simulink library "blocklib"  (R2019b)
settings: Solver=VariableStepAuto  StartTime=0.0  StopTime=10.0  RelTol=1e-3
undefined symbols (not defined in the file or in its folder): magnitude
libraries: $bdroot x11
settings Model: Creator=Imanol  LastModifiedBy=imanol
settings SFSimCC: CustomCodeUndefinedFunction=UseInterfaceOnly

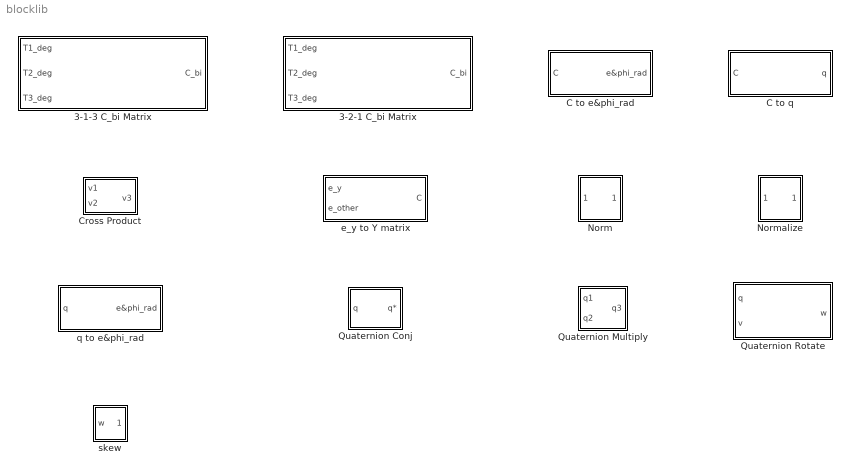
== system blocklib ==
  3-1-3 C_bi Matrix : Subsystem  Tag=|
      | text(.05,.5,'{\itEquation:}  \Sigma \alpha^2 + 
      | \beta^2 \rightarrow \infty, \Pi, \phi_3 = {\bfcool}', 
      | 'hor','left','texmode','on')
      mask Display: text(.5,.5,'R_z^T(\theta_3)\cdot R_x^T(\theta_2)\cdot R_z^T(\theta_1)', 'hor','center','texmode','on')
  3-2-1 C_bi Matrix : Subsystem  Tag=|
      | text(.05,.5,'{\itEquation:}  \Sigma \alpha^2 + 
      | \beta^2 \rightarrow \infty, \Pi, \phi_3 = {\bfcool}', 
      | 'hor','left','texmode','on')
      mask Display: text(.5,.5,'R_x^T(\theta_3)\cdot R_y^T(\theta_2)\cdot R_z^T(\theta_1)', 'hor','center','texmode','on')
  C to e&phi_rad : Subsystem
      mask Display: text(.5,.5,'C\rightarrow [{\bf e}; phi_{rad}]', 'hor','center','texmode','on')
  C to q : Subsystem
      mask Display: text(.5,.5,'C\rightarrow [{\bf q}; q_4]', 'hor','center','texmode','on')
  Cross Product : Subsystem
      mask Display: text(.5,.5,'{\bf v_1} \times {\bf v_2}', 'hor','center','texmode','on')
  Norm : Subsystem
      mask Display: text(.5,.5,'|{\bf u}|', 'hor','center','texmode','on')
  Normalize : Subsystem
      mask Display: text(.5,.5,'{\bf u}/|{\bf u}|', 'hor','center','texmode','on')
  Quaternion Conj : Subsystem
      mask Display: text(.5,.5,'Conj(q)', 'hor','center','texmode','on')
  Quaternion Multiply : Subsystem
      mask Display: text(.5,.5,'q_1\times q_2', 'hor','center','texmode','on')
  Quaternion Rotate : Subsystem
      mask Display: text(.5,.5,'q \times [{\bf v}; 0] \times q^*', 'hor','center','texmode','on')
  e_y to Y matrix : Subsystem
      mask Display: text(.5,.5,'[0;1;0]=C\cdot{\bf e_y}','hor','center', 'texmode','on')
  q to e&phi_rad : Subsystem
      mask Display: text(.5,.5,'q\rightarrow [{\bf e}; phi_{rad}]', 'hor','center','texmode','on')
  skew : Subsystem
      mask Display: text(.5,.5,'w^x', 'hor','center','texmode','on')

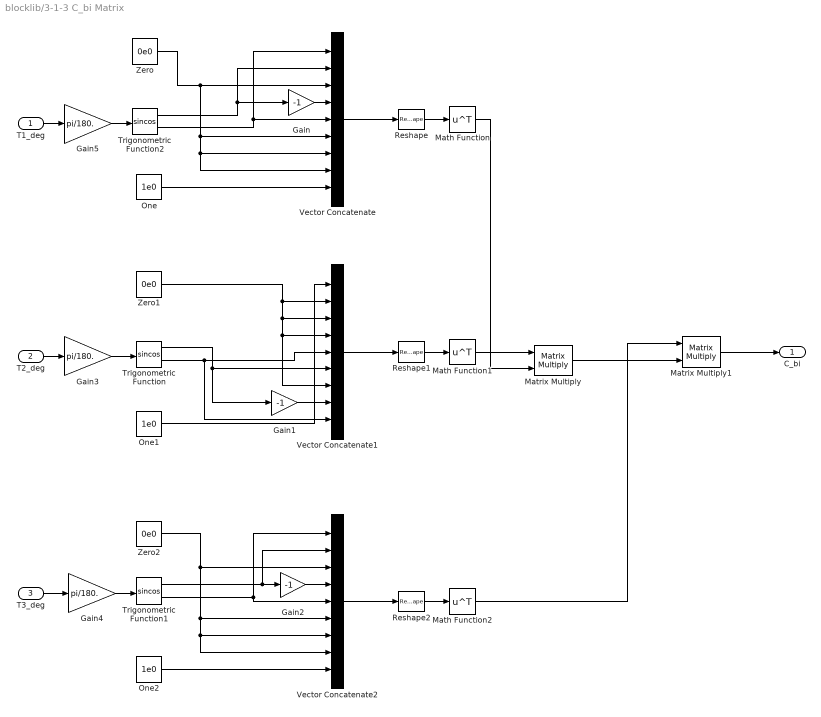
== system blocklib/3-1-3 C_bi Matrix ==
  T1_deg : Inport
  T2_deg : Inport  Port=2
  T3_deg : Inport  Port=3
  Gain : Gain  Gain=-1
  Gain1 : Gain  Gain=-1
  Gain2 : Gain  Gain=-1
  Gain3 : Gain  Gain=pi/180.
  Gain4 : Gain  Gain=pi/180.
  Gain5 : Gain  Gain=pi/180.
  Math Function : Math  Operator=transpose  SignedPower=off  SaturateOnIntegerOverflow=on
  Math Function1 : Math  Operator=transpose  SignedPower=off  SaturateOnIntegerOverflow=on
  Math Function2 : Math  Operator=transpose  SignedPower=off  SaturateOnIntegerOverflow=on
  Matrix Multiply : Product  Multiplication=Matrix(*)
  Matrix Multiply1 : Product  Multiplication=Matrix(*)
  One : Constant  Value=1e0
  One1 : Constant  Value=1e0
  One2 : Constant  Value=1e0
  Reshape : Reshape  OutputDimensionality=Customize  OutputDimensions=[3,3]
  Reshape1 : Reshape  OutputDimensionality=Customize  OutputDimensions=[3,3]
  Reshape2 : Reshape  OutputDimensionality=Customize  OutputDimensions=[3,3]
  Trigonometric Function : Trigonometry  Operator=sincos
  Trigonometric Function1 : Trigonometry  Operator=sincos
  Trigonometric Function2 : Trigonometry  Operator=sincos
  Vector Concatenate : Concatenate  NumInputs=9
  Vector Concatenate1 : Concatenate  NumInputs=9
  Vector Concatenate2 : Concatenate  NumInputs=9
  Zero : Constant  Value=0e0
  Zero1 : Constant  Value=0e0
  Zero2 : Constant  Value=0e0
  C_bi : Outport
  wires:
  T3_deg/1 -> Gain4/1
  T2_deg/1 -> Gain3/1
  Trigonometric Function2/2 -> Vector Concatenate/5, Vector Concatenate/1
  Trigonometric Function2/1 -> Gain/1, Vector Concatenate/2
  Zero/1 -> Vector Concatenate/7, Vector Concatenate/8, Vector Concatenate/6, Vector Concatenate/3
  Gain/1 -> Vector Concatenate/4
  One/1 -> Vector Concatenate/9
  Vector Concatenate/1 -> Reshape/1
  Vector Concatenate1/1 -> Reshape1/1
  One1/1 -> Vector Concatenate1/1
  Zero1/1 -> Vector Concatenate1/7, Vector Concatenate1/4, Vector Concatenate1/3, Vector Concatenate1/2
  Trigonometric Function/2 -> Vector Concatenate1/9, Vector Concatenate1/5
  Trigonometric Function/1 -> Gain1/1, Vector Concatenate1/6
  Gain1/1 -> Vector Concatenate1/8
  Trigonometric Function1/1 -> Vector Concatenate2/2, Gain2/1
  One2/1 -> Vector Concatenate2/9
  Gain2/1 -> Vector Concatenate2/4
  Trigonometric Function1/2 -> Vector Concatenate2/5, Vector Concatenate2/1
  Zero2/1 -> Vector Concatenate2/7, Vector Concatenate2/8, Vector Concatenate2/6, Vector Concatenate2/3
  Reshape1/1 -> Math Function1/1
  Reshape/1 -> Math Function/1
  Matrix Multiply/1 -> Matrix Multiply1/2
  Reshape2/1 -> Math Function2/1
  Matrix Multiply1/1 -> C_bi/1
  Vector Concatenate2/1 -> Reshape2/1
  Gain4/1 -> Trigonometric Function1/1
  Gain3/1 -> Trigonometric Function/1
  T1_deg/1 -> Gain5/1
  Gain5/1 -> Trigonometric Function2/1
  Math Function/1 -> Matrix Multiply/2
  Math Function1/1 -> Matrix Multiply/1
  Math Function2/1 -> Matrix Multiply1/1

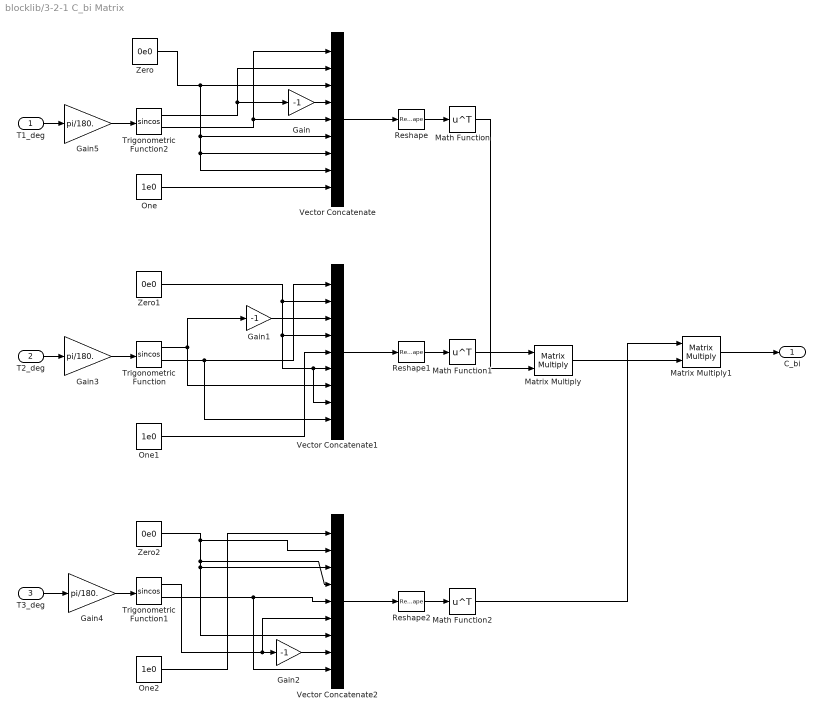
== system blocklib/3-2-1 C_bi Matrix ==
  T1_deg : Inport
  T2_deg : Inport  Port=2
  T3_deg : Inport  Port=3
  Gain : Gain  Gain=-1
  Gain1 : Gain  Gain=-1
  Gain2 : Gain  Gain=-1
  Gain3 : Gain  Gain=pi/180.
  Gain4 : Gain  Gain=pi/180.
  Gain5 : Gain  Gain=pi/180.
  Math Function : Math  Operator=transpose  SignedPower=off  SaturateOnIntegerOverflow=on
  Math Function1 : Math  Operator=transpose  SignedPower=off  SaturateOnIntegerOverflow=on
  Math Function2 : Math  Operator=transpose  SignedPower=off  SaturateOnIntegerOverflow=on
  Matrix Multiply : Product  Multiplication=Matrix(*)
  Matrix Multiply1 : Product  Multiplication=Matrix(*)
  One : Constant  Value=1e0
  One1 : Constant  Value=1e0
  One2 : Constant  Value=1e0
  Reshape : Reshape  OutputDimensionality=Customize  OutputDimensions=[3,3]
  Reshape1 : Reshape  OutputDimensionality=Customize  OutputDimensions=[3,3]
  Reshape2 : Reshape  OutputDimensionality=Customize  OutputDimensions=[3,3]
  Trigonometric Function : Trigonometry  Operator=sincos
  Trigonometric Function1 : Trigonometry  Operator=sincos
  Trigonometric Function2 : Trigonometry  Operator=sincos
  Vector Concatenate : Concatenate  NumInputs=9
  Vector Concatenate1 : Concatenate  NumInputs=9
  Vector Concatenate2 : Concatenate  NumInputs=9
  Zero : Constant  Value=0e0
  Zero1 : Constant  Value=0e0
  Zero2 : Constant  Value=0e0
  C_bi : Outport
  wires:
  T3_deg/1 -> Gain4/1
  T2_deg/1 -> Gain3/1
  Trigonometric Function2/2 -> Vector Concatenate/5, Vector Concatenate/1
  Trigonometric Function2/1 -> Gain/1, Vector Concatenate/2
  Zero/1 -> Vector Concatenate/7, Vector Concatenate/8, Vector Concatenate/6, Vector Concatenate/3
  Gain/1 -> Vector Concatenate/4
  One/1 -> Vector Concatenate/9
  Vector Concatenate/1 -> Reshape/1
  Vector Concatenate1/1 -> Reshape1/1
  One1/1 -> Vector Concatenate1/5
  Zero1/1 -> Vector Concatenate1/2, Vector Concatenate1/8, Vector Concatenate1/6, Vector Concatenate1/4
  Trigonometric Function/2 -> Vector Concatenate1/1, Vector Concatenate1/9
  Trigonometric Function/1 -> Gain1/1, Vector Concatenate1/7
  Gain1/1 -> Vector Concatenate1/3
  Trigonometric Function1/1 -> Vector Concatenate2/6, Gain2/1
  One2/1 -> Vector Concatenate2/1
  Gain2/1 -> Vector Concatenate2/8
  Trigonometric Function1/2 -> Vector Concatenate2/9, Vector Concatenate2/5
  Zero2/1 -> Vector Concatenate2/2, Vector Concatenate2/7, Vector Concatenate2/3, Vector Concatenate2/4
  Reshape1/1 -> Math Function1/1
  Reshape/1 -> Math Function/1
  Matrix Multiply/1 -> Matrix Multiply1/2
  Reshape2/1 -> Math Function2/1
  Matrix Multiply1/1 -> C_bi/1
  Vector Concatenate2/1 -> Reshape2/1
  Gain4/1 -> Trigonometric Function1/1
  Gain3/1 -> Trigonometric Function/1
  T1_deg/1 -> Gain5/1
  Math Function/1 -> Matrix Multiply/2
  Math Function1/1 -> Matrix Multiply/1
  Math Function2/1 -> Matrix Multiply1/1
  Gain5/1 -> Trigonometric Function2/1

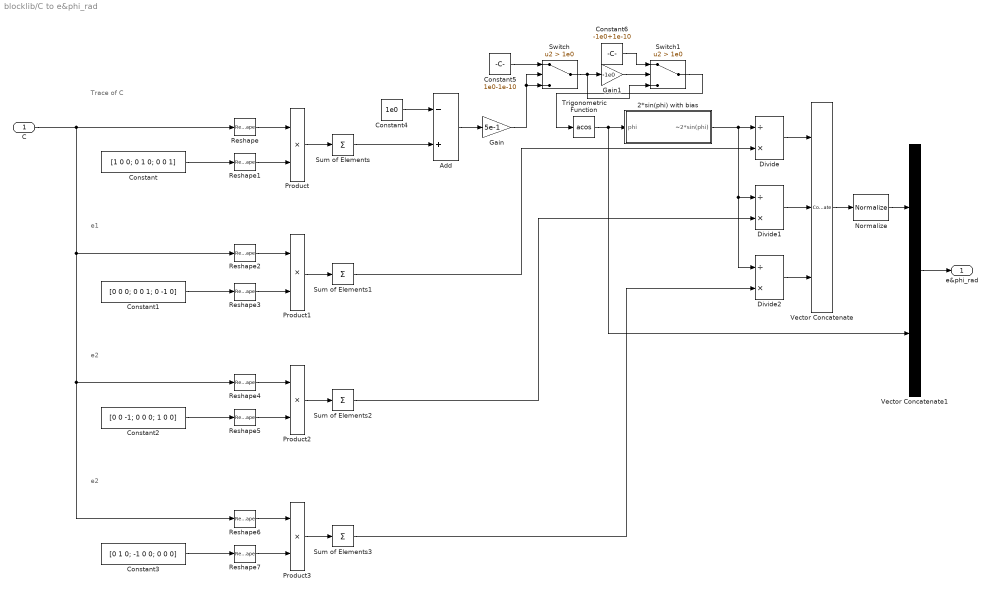
== system blocklib/C to e&phi_rad ==
  note: Trace of C
  note: e1
  note: e2
  note: e2
  C : Inport
  2*sin(phi) with bias : Subsystem
  Add : Sum  Inputs=-+
  Constant : Constant  Value=[1 0 0; 0 1 0; 0 0 1]
  Constant1 : Constant  Value=[0 0 0; 0 0 1; 0 -1 0]
  Constant2 : Constant  Value=[0 0 -1; 0 0 0; 1 0 0]
  Constant3 : Constant  Value=[0 1 0; -1 0 0; 0 0 0]
  Constant4 : Constant  Value=1e0
  Constant5 : Constant  Value=1e0-1e-10
  Constant6 : Constant  Value=-1e0+1e-10
  Divide : Product  Inputs=/*
  Divide1 : Product  Inputs=/*
  Divide2 : Product  Inputs=/*
  Gain : Gain  Gain=5e-1
  Gain1 : Gain  Gain=-1e0
  Normalize : $bdroot/Normalize  SystemSampleTime=-1  Latency=0  AutoFrameSizeCalculation=off
  Product{,1..3} (4 alike) : Product
  Reshape{,1..7} (8 alike) : Reshape  OutputDimensionality=Customize  OutputDimensions=[9,1]
  Sum of Elements{,1..3} (4 alike) : Sum  Inputs=+
  Switch : Switch  Criteria=u2 > Threshold  Threshold=1e0  ZeroCross=off
  Switch1 : Switch  Criteria=u2 > Threshold  Threshold=1e0  ZeroCross=off
  Trigonometric Function : Trigonometry  Operator=acos  OutputSignalType=real
  Vector Concatenate : Concatenate  NumInputs=3
  Vector Concatenate1 : Concatenate
  e&phi_rad : Outport
  wires:
  Switch1/1 -> Trigonometric Function/1
  Constant6/1 -> Switch1/1
  Switch/1 -> Gain1/1, Switch1/3
  Gain1/1 -> Switch1/2
  Constant5/1 -> Switch/1
  Gain/1 -> Switch/2, Switch/3
  Constant/1 -> Reshape1/1
  Reshape1/1 -> Product/2
  Reshape/1 -> Product/1
  Product/1 -> Sum of Elements/1
  Reshape2/1 -> Product1/1
  Product1/1 -> Sum of Elements1/1
  Constant1/1 -> Reshape3/1
  Reshape3/1 -> Product1/2
  Reshape5/1 -> Product2/2
  Constant2/1 -> Reshape5/1
  Product2/1 -> Sum of Elements2/1
  Reshape4/1 -> Product2/1
  Reshape7/1 -> Product3/2
  Reshape6/1 -> Product3/1
  Constant3/1 -> Reshape7/1
  C/1 -> Reshape6/1, Reshape4/1, Reshape2/1, Reshape/1
  Product3/1 -> Sum of Elements3/1
  Sum of Elements/1 -> Add/2
  Constant4/1 -> Add/1
  Add/1 -> Gain/1
  Sum of Elements1/1 -> Divide/2
  Sum of Elements2/1 -> Divide1/2
  Sum of Elements3/1 -> Divide2/2
  Divide/1 -> Vector Concatenate/1
  Divide1/1 -> Vector Concatenate/2
  Divide2/1 -> Vector Concatenate/3
  2*sin(phi) with bias/1(~2*sin(phi)) -> Divide/1, Divide2/1, Divide1/1
  Vector Concatenate1/1 -> e&phi_rad/1
  Vector Concatenate/1 -> Normalize/1
  Trigonometric Function/1 -> Vector Concatenate1/2, 2*sin(phi) with bias/1(phi)
  Normalize/1 -> Vector Concatenate1/1

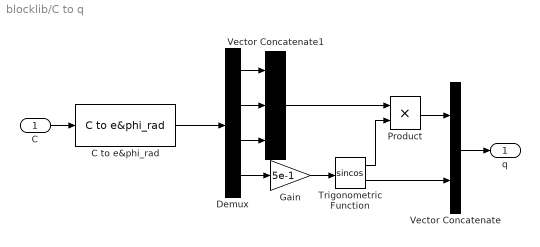
== system blocklib/C to q ==
  C : Inport
  C to e&phi_rad : $bdroot/C to e&phi_rad  SystemSampleTime=-1  Latency=0  AutoFrameSizeCalculation=off
  Demux : Demux
  Gain : Gain  Gain=5e-1
  Product : Product
  Trigonometric Function : Trigonometry  Operator=sincos
  Vector Concatenate : Concatenate
  Vector Concatenate1 : Concatenate  NumInputs=3
  q : Outport
  wires:
  Trigonometric Function/2 -> Vector Concatenate/2
  Demux/3 -> Vector Concatenate1/3
  Demux/4 -> Gain/1
  Demux/2 -> Vector Concatenate1/2
  Vector Concatenate1/1 -> Product/1
  Demux/1 -> Vector Concatenate1/1
  Trigonometric Function/1 -> Product/2
  Product/1 -> Vector Concatenate/1
  Vector Concatenate/1 -> q/1
  Gain/1 -> Trigonometric Function/1
  C/1 -> C to e&phi_rad/1
  C to e&phi_rad/1 -> Demux/1

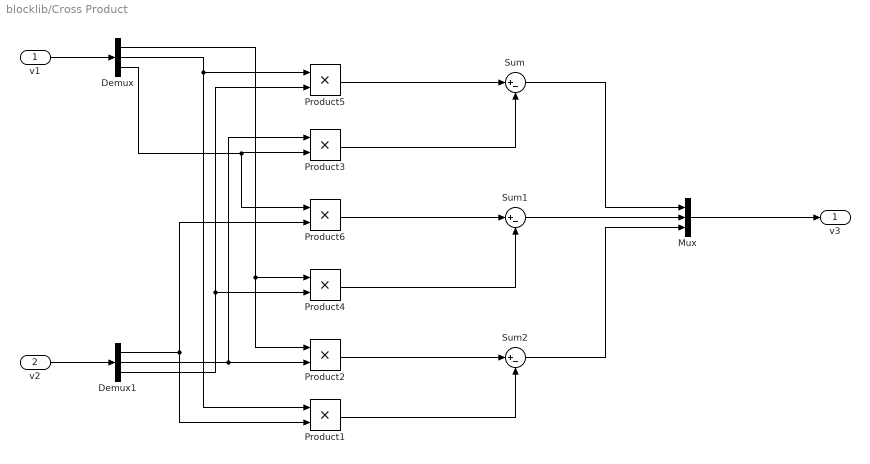
== system blocklib/Cross Product ==
  v1 : Inport
  v2 : Inport  Port=2
  Demux : Demux  Outputs=3
  Demux1 : Demux  Outputs=3
  Mux : Mux  Inputs=3
  Product{1..6} (6 alike) : Product
  Sum : Sum  Inputs=|+-
  Sum1 : Sum  Inputs=|+-
  Sum2 : Sum  Inputs=|+-
  v3 : Outport  VectorParamsAs1DForOutWhenUnconnected=off
  wires:
  Demux/3 -> Product6/1, Product3/2
  Product1/1 -> Sum2/2
  Product2/1 -> Sum2/1
  Product3/1 -> Sum/2
  v2/1 -> Demux1/1
  Demux/2 -> Product1/1, Product5/1
  Demux/1 -> Product2/1, Product4/1
  Product5/1 -> Sum/1
  Demux1/3 -> Product5/2, Product4/2
  Product4/1 -> Sum1/2
  Sum1/1 -> Mux/2
  Sum2/1 -> Mux/3
  v1/1 -> Demux/1
  Demux1/1 -> Product6/2, Product1/2
  Product6/1 -> Sum1/1
  Mux/1 -> v3/1
  Sum/1 -> Mux/1
  Demux1/2 -> Product3/1, Product2/2

== system blocklib/Norm ==
  In1 : Inport
  Math Function : Math  Operator=magnitude^2  SignedPower=off  SaturateOnIntegerOverflow=on
  Sqrt : Sqrt  SaturateOnIntegerOverflow=on
  Sum of Elements : Sum  Inputs=+
  Out1 : Outport
  wires:
  In1/1 -> Math Function/1
  Sum of Elements/1 -> Sqrt/1
  Math Function/1 -> Sum of Elements/1
  Sqrt/1 -> Out1/1

== system blocklib/Normalize ==
  In1 : Inport
  Divide : Product  Inputs=*/
  Math Function : Math  Operator=magnitude^2  SignedPower=off  SaturateOnIntegerOverflow=on
  One : Constant
  Sqrt : Sqrt  SaturateOnIntegerOverflow=on
  Sum of Elements : Sum  Inputs=+
  Switch : Switch  Criteria=u2 > Threshold
  Out1 : Outport
  wires:
  In1/1 -> Divide/1, Math Function/1
  Sqrt/1 -> Switch/1, Switch/2
  Sum of Elements/1 -> Sqrt/1
  Math Function/1 -> Sum of Elements/1
  Divide/1 -> Out1/1
  Switch/1 -> Divide/2
  One/1 -> Switch/3

== system blocklib/Quaternion Conj ==
  q : Inport
  Demux1 : Demux
  Gain : Gain  Gain=-1e0
  Mux1 : Mux  Inputs=3
  Vector Concatenate : Concatenate
  q* : Outport  VectorParamsAs1DForOutWhenUnconnected=off
  wires:
  q/1 -> Demux1/1
  Demux1/1 -> Mux1/1
  Demux1/2 -> Mux1/2
  Demux1/3 -> Mux1/3
  Mux1/1 -> Gain/1
  Gain/1 -> Vector Concatenate/1
  Vector Concatenate/1 -> q*/1
  Demux1/4 -> Vector Concatenate/2

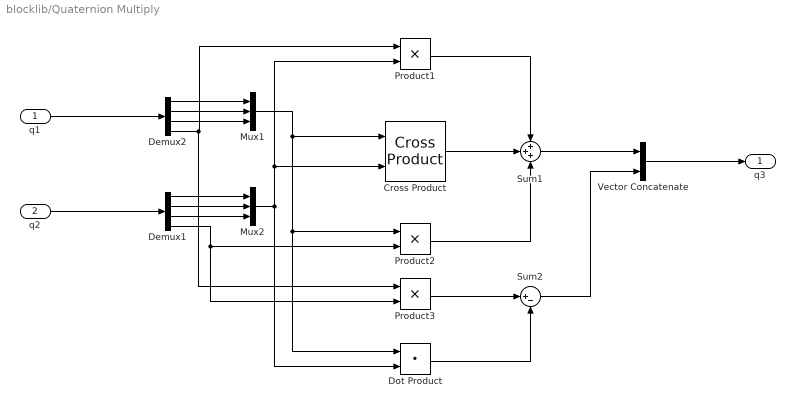
== system blocklib/Quaternion Multiply ==
  q1 : Inport
  q2 : Inport  Port=2
  Cross Product : $bdroot/Cross Product  SystemSampleTime=-1  Latency=0  AutoFrameSizeCalculation=off
  Demux1 : Demux
  Demux2 : Demux
  Dot Product : DotProduct  InputSameDT=on  OutDataTypeStr=Inherit: Inherit via internal rule
  Mux1 : Mux  Inputs=3
  Mux2 : Mux  Inputs=3
  Product1 : Product
  Product2 : Product
  Product3 : Product
  Sum1 : Sum  Inputs=+++
  Sum2 : Sum  Inputs=|+-
  Vector Concatenate : Concatenate
  q3 : Outport  VectorParamsAs1DForOutWhenUnconnected=off
  wires:
  Demux2/3 -> Mux1/3
  Product2/1 -> Sum1/3
  Demux2/2 -> Mux1/2
  Demux1/2 -> Mux2/2
  Mux2/1 -> Product1/2, Cross Product/2, Dot Product/2
  Mux1/1 -> Cross Product/1, Dot Product/1, Product2/1
  Demux1/3 -> Mux2/3
  Demux1/1 -> Mux2/1
  Demux2/4 -> Product3/1, Product1/1
  Demux1/4 -> Product3/2, Product2/2
  Cross Product/1 -> Sum1/2
  Demux2/1 -> Mux1/1
  Product3/1 -> Sum2/1
  q2/1 -> Demux1/1
  Sum2/1 -> Vector Concatenate/2
  Dot Product/1 -> Sum2/2
  Product1/1 -> Sum1/1
  Sum1/1 -> Vector Concatenate/1
  q1/1 -> Demux2/1
  Vector Concatenate/1 -> q3/1

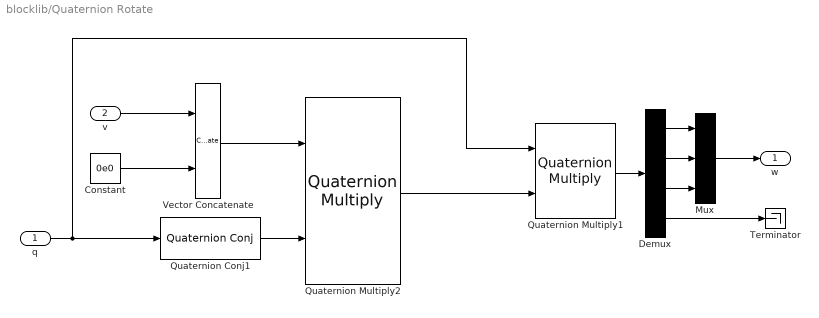
== system blocklib/Quaternion Rotate ==
  q : Inport
  v : Inport  Port=2
  Constant : Constant  Value=0e0
  Demux : Demux
  Mux : Mux  Inputs=3
  Quaternion Conj1 : $bdroot/Quaternion Conj  SystemSampleTime=-1  Latency=0  AutoFrameSizeCalculation=off
  Quaternion Multiply1 : $bdroot/Quaternion Multiply  SystemSampleTime=-1  Latency=0  AutoFrameSizeCalculation=off
  Quaternion Multiply2 : $bdroot/Quaternion Multiply  SystemSampleTime=-1  Latency=0  AutoFrameSizeCalculation=off
  Terminator : Terminator
  Vector Concatenate : Concatenate
  w : Outport  VectorParamsAs1DForOutWhenUnconnected=off
  wires:
  v/1 -> Vector Concatenate/1
  Constant/1 -> Vector Concatenate/2
  q/1 -> Quaternion Conj1/1, Quaternion Multiply1/1
  Vector Concatenate/1 -> Quaternion Multiply2/1
  Quaternion Conj1/1 -> Quaternion Multiply2/2
  Quaternion Multiply2/1 -> Quaternion Multiply1/2
  Quaternion Multiply1/1 -> Demux/1
  Demux/1 -> Mux/1
  Demux/2 -> Mux/2
  Demux/3 -> Mux/3
  Mux/1 -> w/1
  Demux/4 -> Terminator/1

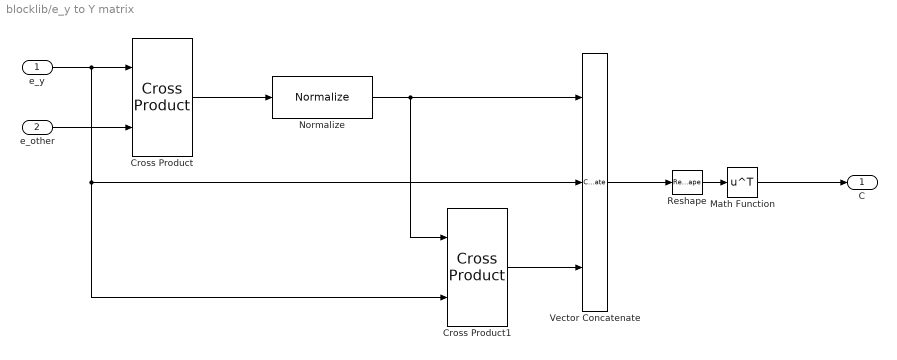
== system blocklib/e_y to Y matrix ==
  e_y : Inport
  e_other : Inport  Port=2
  Cross Product : $bdroot/Cross Product  SystemSampleTime=-1  Latency=0  AutoFrameSizeCalculation=off
  Cross Product1 : $bdroot/Cross Product  SystemSampleTime=-1  Latency=0  AutoFrameSizeCalculation=off
  Math Function : Math  Operator=transpose  SignedPower=off  SaturateOnIntegerOverflow=on
  Normalize : $bdroot/Normalize  SystemSampleTime=-1  Latency=0  AutoFrameSizeCalculation=off
  Reshape : Reshape  OutputDimensionality=Customize  OutputDimensions=[3,3]
  Vector Concatenate : Concatenate  NumInputs=3
  C : Outport
  wires:
  e_other/1 -> Cross Product/2
  e_y/1 -> Vector Concatenate/2, Cross Product1/2, Cross Product/1
  Cross Product/1 -> Normalize/1
  Normalize/1 -> Cross Product1/1, Vector Concatenate/1
  Cross Product1/1 -> Vector Concatenate/3
  Vector Concatenate/1 -> Reshape/1
  Reshape/1 -> Math Function/1
  Math Function/1 -> C/1

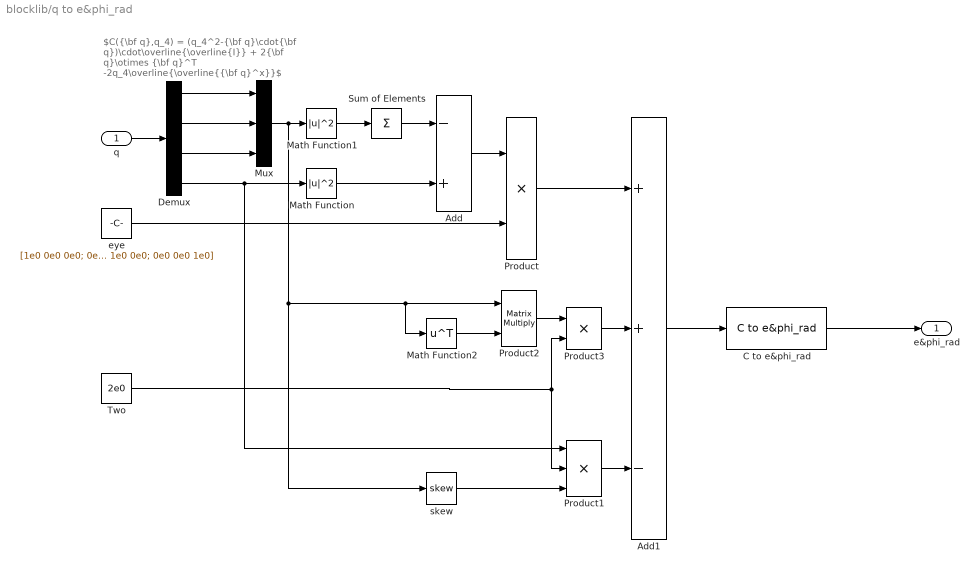
== system blocklib/q to e&phi_rad ==
  note: $C({\bf q},q_4) = (q_4^2-{\bf q}\cdot{\bf q})\cdot\overline{\overline{I}} + 2{\bf q}\otimes {\bf q}^T -2q_4\overline{\overline{{\bf q}^x}}$
  q : Inport
  Add : Sum  Inputs=-+
  Add1 : Sum  Inputs=++-
  C to e&phi_rad : $bdroot/C to e&phi_rad  SystemSampleTime=-1  Latency=0  AutoFrameSizeCalculation=off
  Demux : Demux
  Math Function : Math  Operator=magnitude^2  SignedPower=off  SaturateOnIntegerOverflow=on
  Math Function1 : Math  Operator=magnitude^2  SignedPower=off  SaturateOnIntegerOverflow=on
  Math Function2 : Math  Operator=transpose  SignedPower=off  SaturateOnIntegerOverflow=on
  Mux : Mux  Inputs=3
  Product : Product
  Product1 : Product  Inputs=3
  Product2 : Product  Multiplication=Matrix(*)
  Product3 : Product
  Sum of Elements : Sum  Inputs=+
  Two : Constant  Value=2e0
  eye : Constant  Value=[1e0 0e0 0e0; 0e0 1e0 0e0; 0e0 0e0 1e0]
  skew : $bdroot/skew  SystemSampleTime=-1  Latency=0  AutoFrameSizeCalculation=off
  e&phi_rad : Outport
  wires:
  Product1/1 -> Add1/3
  Product2/1 -> Product3/1
  Product3/1 -> Add1/2
  C to e&phi_rad/1 -> e&phi_rad/1
  q/1 -> Demux/1
  Demux/1 -> Mux/1
  Demux/2 -> Mux/2
  Demux/3 -> Mux/3
  Demux/4 -> Math Function/1, Product1/1
  Mux/1 -> Math Function2/1, Product2/1, skew/1, Math Function1/1
  Math Function1/1 -> Sum of Elements/1
  Sum of Elements/1 -> Add/1
  Math Function/1 -> Add/2
  Add/1 -> Product/1
  eye/1 -> Product/2
  Product/1 -> Add1/1
  Add1/1 -> C to e&phi_rad/1
  Two/1 -> Product3/2, Product1/2
  skew/1 -> Product1/3
  Math Function2/1 -> Product2/2

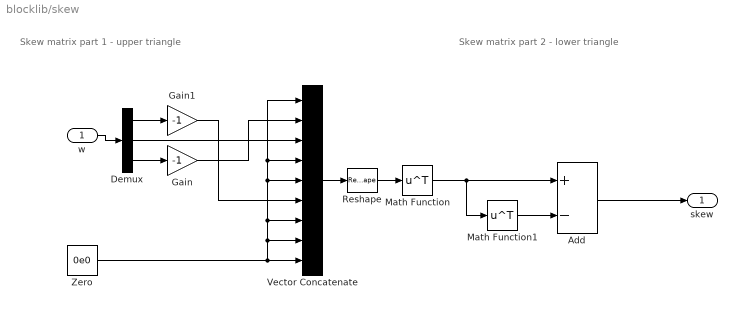
== system blocklib/skew ==
  note: Skew matrix part 2 - lower triangle
  note: Skew matrix part 1 - upper triangle
  w : Inport
  Add : Sum  Inputs=+-
  Demux : Demux  Outputs=3
  Gain : Gain  Gain=-1
  Gain1 : Gain  Gain=-1
  Math Function : Math  Operator=transpose  SignedPower=off  SaturateOnIntegerOverflow=on
  Math Function1 : Math  Operator=transpose  SignedPower=off  SaturateOnIntegerOverflow=on
  Reshape : Reshape  OutputDimensionality=Customize  OutputDimensions=[3,3]
  Vector Concatenate : Concatenate  NumInputs=9
  Zero : Constant  Value=0e0
  skew : Outport
  wires:
  Reshape/1 -> Math Function/1
  w/1 -> Demux/1
  Zero/1 -> Vector Concatenate/4, Vector Concatenate/1, Vector Concatenate/5, Vector Concatenate/7, Vector Concatenate/8, Vector Concatenate/9
  Demux/1 -> Gain1/1
  Demux/3 -> Gain/1
  Gain/1 -> Vector Concatenate/2
  Demux/2 -> Vector Concatenate/3
  Gain1/1 -> Vector Concatenate/6
  Vector Concatenate/1 -> Reshape/1
  Math Function/1 -> Math Function1/1, Add/1
  Add/1 -> skew/1
  Math Function1/1 -> Add/2

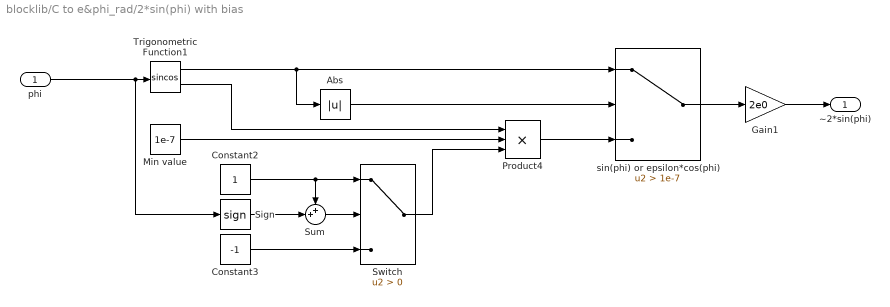
== system blocklib/C to e&phi_rad/2*sin(phi) with bias ==
  phi : Inport
  Abs : Abs
  Constant2 : Constant
  Constant3 : Constant  Value=-1
  Gain1 : Gain  Gain=2e0
  Min value : Constant  Value=1e-7
  Product4 : Product  Inputs=3
  Sign : Signum  ZeroCross=off
  Sum : Sum  Inputs=++|
  Switch : Switch  Criteria=u2 > Threshold  ZeroCross=off
  Trigonometric Function1 : Trigonometry  Operator=sincos
  sin(phi) or epsilon*cos(phi) : Switch  Criteria=u2 > Threshold  Threshold=1e-7  ZeroCross=off
  ~2*sin(phi) : Outport
  wires:
  Abs/1 -> sin(phi) or epsilon*cos(phi)/2
  Trigonometric Function1/1 -> Abs/1, sin(phi) or epsilon*cos(phi)/1
  Trigonometric Function1/2 -> Product4/1
  Min value/1 -> Product4/2
  sin(phi) or epsilon*cos(phi)/1 -> Gain1/1
  phi/1 -> Sign/1, Trigonometric Function1/1
  Gain1/1 -> ~2*sin(phi)/1
  Product4/1 -> sin(phi) or epsilon*cos(phi)/3
  Switch/1 -> Product4/3
  Constant3/1 -> Switch/3
  Constant2/1 -> Sum/1, Switch/1
  Sum/1 -> Switch/2
  Sign/1 -> Sum/2
